simulink model "segmentB_logic"  (R2017a)
settings: Solver=FixedStepDiscrete  StartTime=0.0  StopTime=inf  FixedStep=0.01  RelTol=1e-3
PreLoadFcn:
  | robotParameters;
  | load examplePathNavigationMap.mat;
undefined symbols (not defined in the file or in its folder): motorIp, motorSp
libraries: mobileRoboticsTrainingLib x5
settings Model: Creator=sseshadr  LastModifiedBy=shiremat

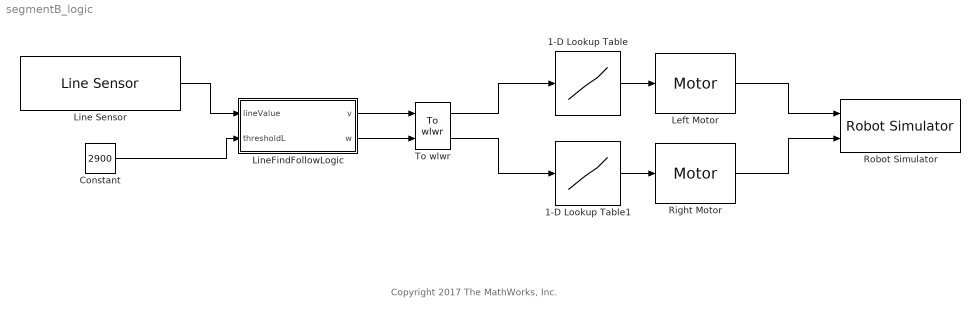
== system segmentB_logic ==
  note: Copyright 2017 The MathWorks, Inc.
  1-D Lookup Table : Lookup_n-D  NumberOfTableDimensions=1  BreakpointsForDimension1=motorSp  Table=motorIp  ExtrapMethod=Clip  InternalRulePriority=Speed  RndMeth=Simplest  InputSameDT=on
  1-D Lookup Table1 : Lookup_n-D  NumberOfTableDimensions=1  BreakpointsForDimension1=motorSp  Table=motorIp  ExtrapMethod=Clip  InternalRulePriority=Speed  RndMeth=Simplest  InputSameDT=on
  Constant : Constant  Value=2900
  Left Motor : mobileRoboticsTrainingLib/Motor  motorPlant=wheelMotorModel  sensorType=Speed
      settings: SourceProductName=Mobile Robotics Training Library
  Line Sensor : mobileRoboticsTrainingLib/Line Sensor  mapVariable=mapForSim  envVal=2850  lineVal=2950  sensOff=[0.01 -0.01;0.01 0;0.01 0.01]
      settings: SourceProductName=Mobile Robotics Training Library
  LineFindFollowLogic : Stateflow chart  TreatAsAtomicUnit=on
  Right Motor : mobileRoboticsTrainingLib/Motor  motorPlant=wheelMotorModel  sensorType=Speed
      settings: SourceProductName=Mobile Robotics Training Library
  Robot Simulator : mobileRoboticsTrainingLib/Robot Simulator  Priority=99  mapVar=mapForSim  startX=0.59375  startY=1.26  startTheta=-4  axleLength=axleLength  wheelR=wheelR
  To wlwr : mobileRoboticsTrainingLib/To wlwr  axleLength=axleLength  wheelR=wheelR
  wires:
  Left Motor/1 -> Robot Simulator/1
  1-D Lookup Table1/1 -> Right Motor/1
  1-D Lookup Table/1 -> Left Motor/1
  Right Motor/1 -> Robot Simulator/2
  To wlwr/1 -> 1-D Lookup Table/1
  To wlwr/2 -> 1-D Lookup Table1/1
  LineFindFollowLogic/1(v) -> To wlwr/1
  LineFindFollowLogic/2(w) -> To wlwr/2
  Line Sensor/1 -> LineFindFollowLogic/1(lineValue)
  Constant/1 -> LineFindFollowLogic/2(thresholdL)

== stateflow chart segmentB_logic/LineFindFollowLogic ==
  state FindLine
    entry:
    v = 0.05;
  state GoLeft
    entry:
    v = 0.1;
    w = 1;
  state GoRight
    entry:
    v = 0.1;
    w = -1;
  state Stop
    entry:
    v = 0;
    w = 0;
  (default) -> FindLine
  FindLine -> GoLeft : [lineValue(2) > thresholdL]
  GoLeft -> GoRight [order 1] : [lineValue(2) < thresholdL]
  GoRight -> GoLeft [order 1] : [lineValue(2) >= thresholdL]
  GoLeft -> Stop [order 2] : [all(lineValue > thresholdL)]
  GoRight -> Stop [order 2] : [all(lineValue > thresholdL)]
  data: v output; w output; lineValue input; thresholdL input
